simulink model "File_Demod_rx"  (R2023b)
settings: Solver=FixedStepDiscrete  StartTime=0.0  StopTime=10.0  FixedStep=0.02  RelTol=1e-3
libraries: dspsnks4 x1, dspmlti4 x1, commanabbnd3 x1, dspfdesign x1
settings Model: Creator=123  LastModifiedBy=yuezh

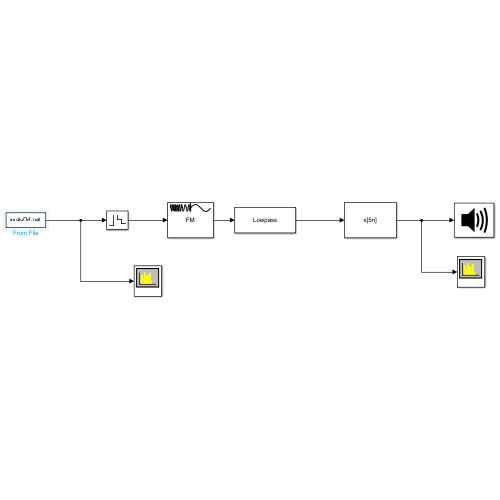
[thumbnail: Simulink's stored preview of the top-level diagram]
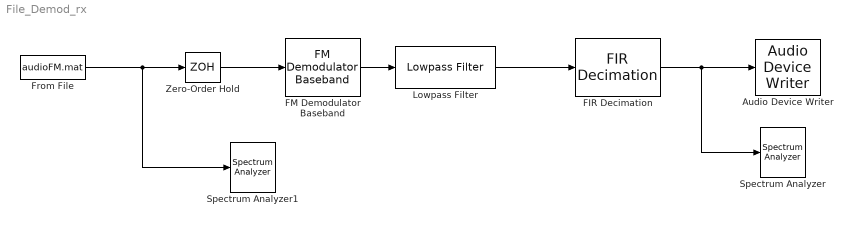
== system File_Demod_rx ==
  Audio Device Writer : dspsnks4/Audio Device Writer  Driver=DirectSound  Device=Default  InheritSampleRate=on  SampleRate=44100  BitDepth=16-bit integer  BufferSize=4096  NumBuffers=10  DefaultOutputChannelMapping=on  OutputChannelMapping=1:2  OutputNumUnderrunSamples=off  DriverIdx=1  DeviceWarnFlag=''
  FIR Decimation : dspmlti4/FIR Decimation  FilterSource=Dialog parameters  h=firpm(100, [0 40e3 60e3 (360e3/2)]/(360e3/2), [1 1 0 0], [1 1], 20)  D=5  filtStruct=Direct form  FilterObject=FDECIM  InputProcessing=Columns as channels (frame based)  framing=Allow multirate processing  AllowArbitraryInputLength=off  inputOffset=0  outputBufInitCond=0  roundingMode=Floor  overflowMode=off  firstCoeffDataTypeStr=Inherit: Same word length as input  firstCoeffMin=[]  firstCoeffMax=[]  firstCoeffLastDataTypeStr=Inherit: Same word length as input  outputDataTypeStr=Inherit: Same as accumulator  outputMin=[]  outputMax=[]  outputLastDataTypeStr=Inherit: Same as accumulator
  "FM Demodulator Baseband " : commanabbnd3/FM Demodulator Baseband   FrequencyDeviation=75e3  SimulateUsing=Code generation
  From File : FromFile  FileName=audioFM.mat  OutDataTypeStr=double  SampleTime=0.02  ExtrapolationBeforeFirstDataPoint=Hold first value  InterpolationWithinTimeRange=Zero order hold  ExtrapolationAfterLastDataPoint=Hold last value
  Lowpass Filter : dspfdesign/Lowpass Filter  FilterType=FIR  DesignForMinimumOrder=on  FilterOrder=50  PassbandFrequency=15e3  StopbandFrequency=20e3  PassbandRipple=0.1  StopbandAttenuation=80  SampleRateMode=Specify on dialog  SampleRate=240e3  SimulateUsing=Interpreted execution  roundingMode=Floor  coeffsDataTypeStr=fixdt(1,16)
  Spectrum Analyzer : SpectrumAnalyzer  WindowPosition=[560.000000,350.000000,800.000000,500.000000,]  ScopeFrameLocation=window  SampleRateSource=Property  SampleRate=44.1e3  PlotAsTwoSidedSpectrum=off  FrequencyScale=Log  FrequencySpan=Start and stop frequencies  StartFrequency=20  StopFrequency=20e3  YLimits=[-168.98171478,13.8252145]
  Spectrum Analyzer1 : SpectrumAnalyzer  WindowPosition=[560.000000,350.000000,800.000000,500.000000,]  ScopeFrameLocation=window  SampleRateSource=Property  SampleRate=44.1e3  PlotAsTwoSidedSpectrum=off  FrequencyScale=Log  FrequencySpan=Start and stop frequencies  StartFrequency=20  StopFrequency=20e3  YLimits=[-177.9020505,36.38002988]
  Zero-Order Hold : ZeroOrderHold  SampleTime=0.02
  wires:
  Lowpass Filter/1 -> FIR Decimation/1
  FIR Decimation/1 -> Spectrum Analyzer/1, Audio Device Writer/1
  "FM Demodulator Baseband "/1 -> Lowpass Filter/1
  From File/1 -> Zero-Order Hold/1, Spectrum Analyzer1/1
  Zero-Order Hold/1 -> "FM Demodulator Baseband "/1
